simulink model "ROSCO"  (R2022b)
settings: Solver=ode4  StartTime=0.0  StopTime=TMax  FixedStep=simu.dt  RelTol=1e-3  EnableMultiTasking=on
undefined symbols (not defined in the file): DiscIntNeverNeededParam, F, OutList, Parameter, R, rpm2radps, simu, strmatch
libraries: simulink x10
(part 1 of 3)
settings Model: Creator=nabbas  LastModifiedBy=emanu
settings SolverCC: AlgebraicLoopSolver=TrustRegion
settings DataIOCC: SaveTime=off  ReturnWorkspaceOutputs=off  SignalLoggingName=sigsOut
settings OptimizationCC: OptimizeBlockIOStorage=off
settings DebuggingCC: UnconnectedInputMsg=warning  UnconnectedOutputMsg=warning  UnconnectedLineMsg=warning  SFMachineParentedDataDiag=warning  ArithmeticOperatorsInVariantConditions=warning
settings ModelReferenceCC: EnableRefExpFcnMdlSchedulingChecks=on
settings SFSimCC: SimUseLocalCustomCode=off  CustomCodeUndefinedFunction=UseInterfaceOnly
settings RTWCC: RTWUseLocalCustomCode=off  BuildConfiguration=Debug
settings CodeAppCC: ForceParamTrailComments=on  StateflowObjectComments=on  MATLABSourceComments=on

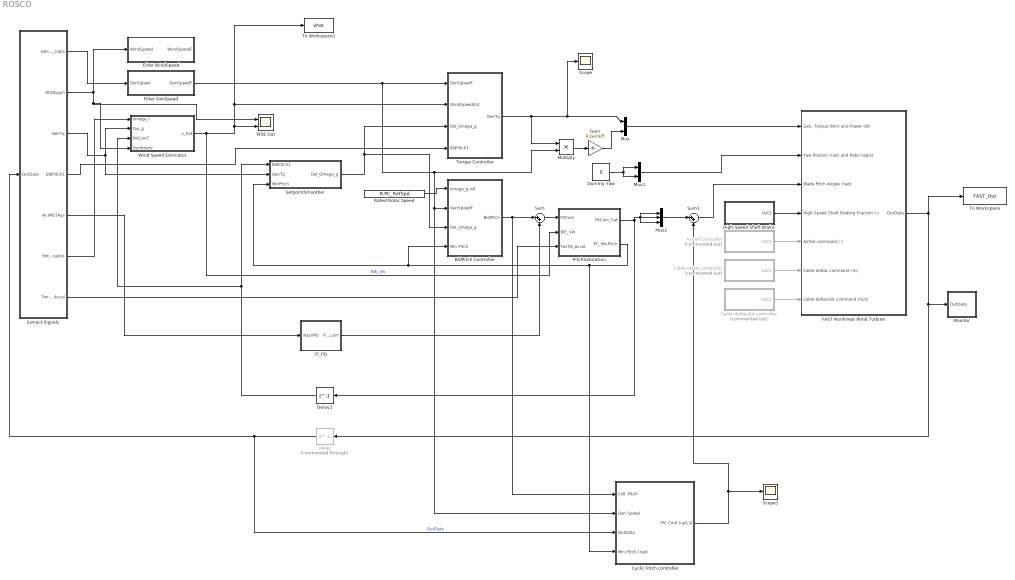
== system ROSCO ==
  AirFoil Controller : Subsystem  Commented=on
  BldPitch Controller : Subsystem
  Cable deltaL controller : Subsystem  Commented=on
  Cable deltaLdot controller : Subsystem  Commented=on
  Cyclic Pitch controller : Subsystem  TreatAsAtomicUnit=on
      settings: MinAlgLoopOccurrences=on
  Delay : Delay  Commented=through  DelayLength=1
  Delay1 : Delay  DelayLength=1
  Dummy Yaw : Constant  Value=0
  Extract Signals : Subsystem  TreatAsAtomicUnit=on
  FAST Nonlinear Wind Turbine : Subsystem  mask(FAST Nonlinear Wind Turbine){}
      mask help: This block contains the FAST S-Function.
      mask init:
      | clear FAST_SFunc
  Filter GenSpeed : Subsystem
  Filter WindSpeed : Subsystem
  Fl_PD : Subsystem
  Gain : Gain  Gain=R.GenEff
  High-Speed Shaft Brake : Subsystem
  Monitor : Subsystem  TreatAsAtomicUnit=on
  Multiply : Product
  Mux : Mux  Inputs=2
  Mux1 : Mux  Inputs=2
  Mux2 : Mux  Inputs=3
  PitchSaturation : Subsystem
  Rated Rotor Speed : Constant  Value=R.PC_RefSpd
  Scope : Scope
  Scope1 : Scope
  SetpointSmoother : Subsystem
  Sum : Sum  Inputs=|++
  Sum1 : Sum  Inputs=|++
  To Workspace : ToWorkspace  VariableName=FAST_Out  SaveFormat=Timeseries  SampleTime=-1
  To Workspace1 : ToWorkspace  VariableName=vhat  SaveFormat=Timeseries  SampleTime=-1
  Torque Controller : Subsystem
  WSE Out : Scope  NumInputPorts=2
  Wind Speed Estimator : Subsystem
  wires:
  FAST Nonlinear Wind Turbine/1(OutData) -> To Workspace/1, Delay/1, Monitor/1(OutData)
  Dummy Yaw/1 -> Mux1/2, Mux1/1
  Mux1/1 -> FAST Nonlinear Wind Turbine/2(Yaw Position (rad) and Rate (rad/s))
  Multiply/1 -> Gain/1
  Extract Signals/1(GenSpeed_rad/s) -> Filter GenSpeed/1(GenSpeed)
  Torque Controller/1(GenTq) -> Scope/1, Mux/1, Multiply/1
  Extract Signals/3(GenTq) -> Wind Speed Estimator/2(tau_g), SetpointSmoother/2(GenTq)
  SetpointSmoother/1(Del_Omega_g) -> BldPitch Controller/3(Del_omega_g), Torque Controller/3(Del_omega_g)
  Rated Rotor Speed/1 -> BldPitch Controller/1(omega_g,ref)
  Gain/1 -> Mux/2
  Extract Signals/2(RtVAvgxh) -> Wind Speed Estimator/4(HorWindV), WSE Out/1, Filter WindSpeed/1(WindSpeed)
  Wind Speed Estimator/1(v_hat) -> PitchSaturation/2(WE_Vw), WSE Out/2, Torque Controller/2(WindSpeedEst), To Workspace1/1  "WE_Vw"
  Delay/1 -> Cyclic Pitch controller/3(OutData), Extract Signals/1(OutData)  "OutData"
  Extract Signals/5(NcIMUTAys) -> Fl_PD/1(NacIMU)
  Fl_PD/1(Fl_Pitcom) -> Sum/2
  Extract Signals/4(BldPitch1) -> Torque Controller/4(BldPitch1)
  Sum/1 -> PitchSaturation/1(PitCom)
  PitchSaturation/1(PitCom_Sat) -> Delay1/1, Mux2/3, Mux2/1, Mux2/2
  PitchSaturation/2(PC_MinPitch) -> Cyclic Pitch controller/4(Min PItch (rad)), BldPitch Controller/4(Min Pitch), SetpointSmoother/3(MinPitch)
  BldPitch Controller/1(BldPitch) -> Cyclic Pitch controller/1(Coll. Pitch), Sum/1
  Extract Signals/6(RotSpeed (rad/s)) -> Wind Speed Estimator/1(omega_r)
  Delay1/1 -> SetpointSmoother/1(BldPitch1), Wind Speed Estimator/3(PitComT)
  Extract Signals/7(TwrFA Accel) -> PitchSaturation/3(TwrFA_Accel)
  Mux/1 -> FAST Nonlinear Wind Turbine/1(Gen. Torque (Nm) and Power (W))
  Filter GenSpeed/1(GenSpeedF) -> Torque Controller/1(GenSpeedF), Multiply/2, BldPitch Controller/2(GenSpeedF), Cyclic Pitch controller/2(Gen Speed)
  Cyclic Pitch controller/1(IPC Cmd (rad,3)) -> Scope1/1, Sum1/2
  Mux2/1 -> Sum1/1
  Sum1/1 -> FAST Nonlinear Wind Turbine/3(Blade Pitch Angles (rad))
  High-Speed Shaft Brake/1(Out1) -> FAST Nonlinear Wind Turbine/4(High-Speed Shaft Braking Fraction (-))
  AirFoil Controller/1(Out1) -> FAST Nonlinear Wind Turbine/5(AirFoil command (-))
  Cable deltaL controller/1(Out1) -> FAST Nonlinear Wind Turbine/6(Cable deltaL command (m))
  Cable deltaLdot controller/1(Out1) -> FAST Nonlinear Wind Turbine/7(Cable deltaLdot command (m/s))

== system ROSCO/AirFoil Controller ==
  Airfoil command : Constant  Value=zeros(1,3)'
  Out1 : Outport
  wires:
  Airfoil command/1 -> Out1/1

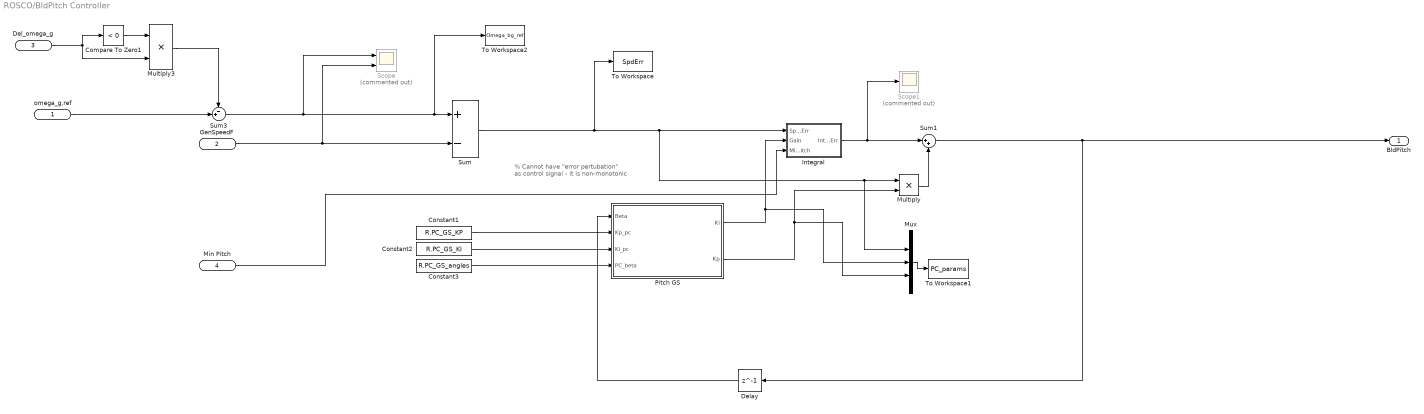
== system ROSCO/BldPitch Controller ==
  note: % Cannot have "error pertubation" as control signal
      | - it is non-monotonic
  omega_g,ref : Inport
  GenSpeedF : Inport  Port=2
  Del_omega_g : Inport  Port=3
  Min Pitch : Inport  Port=4
  Compare To Zero1 : simulink/Logic and Bit Operations/Compare To Zero  relop=<  OutDataTypeStr=boolean
  Constant1 : Constant  Value=R.PC_GS_KP
  Constant2 : Constant  Value=R.PC_GS_KI
  Constant3 : Constant  Value=R.PC_GS_angles
  Delay : Delay  DelayLength=1
  Integral : Subsystem
  Multiply : Product
  Multiply3 : Product
  Mux : Mux  Inputs=5
  Pitch GS : MATLAB Function  TreatAsAtomicUnit=on
  Scope : Scope  Commented=on  NumInputPorts=2
  Scope1 : Scope  Commented=on
  Sum : Sum  Inputs=+-
  Sum1 : Sum  Inputs=|++
  Sum3 : Sum  Inputs=-+|
  To Workspace : ToWorkspace  VariableName=SpdErr  SaveFormat=Timeseries  SampleTime=-1
  To Workspace1 : ToWorkspace  VariableName=PC_params  SaveFormat=Structure  SampleTime=-1
  To Workspace2 : ToWorkspace  VariableName=Omega_bg_ref  SaveFormat=Timeseries  SampleTime=-1
  BldPitch : Outport  VectorParamsAs1DForOutWhenUnconnected=off
  wires:
  Multiply/1 -> Sum1/2
  Integral/1(IntSpdErr) -> Scope1/1, Sum1/1
  Pitch GS/1(Ki) -> Mux/3, Integral/2(Gain)
  Pitch GS/2(Kp) -> Mux/4, Multiply/2
  Mux/1 -> To Workspace1/1
  Sum1/1 -> Delay/1, BldPitch/1
  Sum3/1 -> Scope/1, To Workspace2/1, Sum/1
  GenSpeedF/1 -> Scope/2, Sum/2
  Compare To Zero1/1 -> Multiply3/1
  Del_omega_g/1 -> Compare To Zero1/1, Multiply3/2
  Multiply3/1 -> Sum3/1
  omega_g,ref/1 -> Sum3/2
  Constant1/1 -> Pitch GS/2(Kp_pc)
  Constant2/1 -> Pitch GS/3(Ki_pc)
  Constant3/1 -> Pitch GS/4(PC_beta)
  Delay/1 -> Pitch GS/1(Beta)
  Min Pitch/1 -> Integral/3(Min Pitch)
  Sum/1 -> To Workspace/1, Mux/2, Multiply/1, Integral/1(SpeedErr)

== system ROSCO/Cable deltaL controller ==
  Cable deltaL command : Constant  Value=zeros(1,20)'
  Out1 : Outport
  wires:
  Cable deltaL command/1 -> Out1/1

== system ROSCO/Cable deltaLdot controller ==
  Cable deltaLdot command : Constant  Value=zeros(1,20)'
  Out1 : Outport
  wires:
  Cable deltaLdot command/1 -> Out1/1

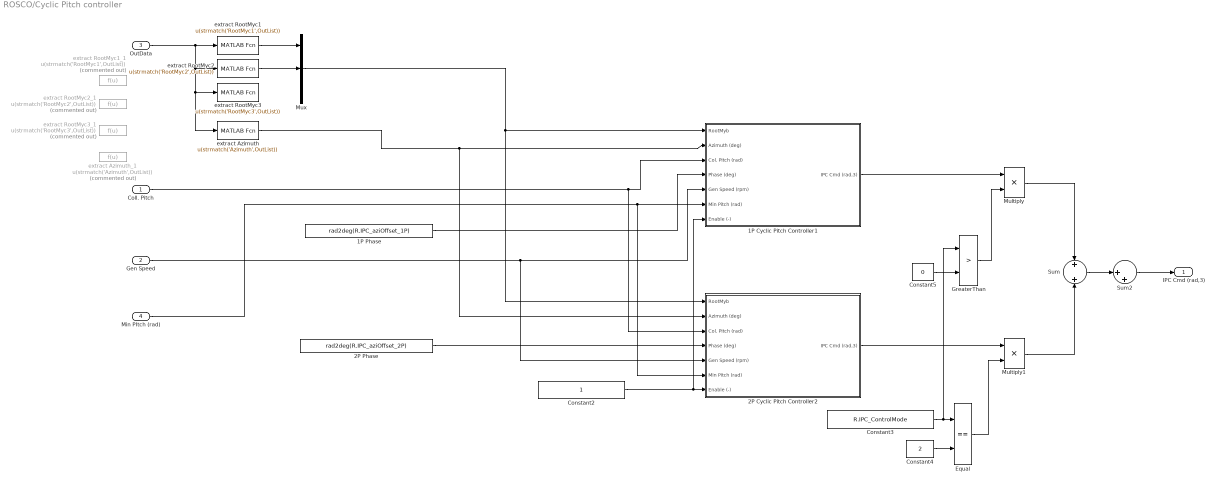
== system ROSCO/Cyclic Pitch controller ==
  Coll. Pitch : Inport
  Gen Speed : Inport  Port=2
  OutData : Inport  Port=3
  Min PItch (rad) : Inport  Port=4
  1P Cyclic Pitch Controller1 : Subsystem
  1P Phase : Constant  Value=rad2deg(R.IPC_aziOffset_1P)
  2P Cyclic Pitch Controller2 : Subsystem
  2P Phase : Constant  Value=rad2deg(R.IPC_aziOffset_2P)
  Constant2 : Constant
  Constant3 : Constant  Value=R.IPC_ControlMode
  Constant4 : Constant  Value=2
  Constant5 : Constant  Value=0
  Equal : RelationalOperator  Operator===  OutDataTypeStr=boolean  RndMeth=Simplest  InputSameDT=off
  GreaterThan : RelationalOperator  Operator=>  OutDataTypeStr=boolean  RndMeth=Simplest  InputSameDT=off
  Multiply : Product
  Multiply1 : Product
  Mux : Mux  Inputs=3
  Sum : Sum  Inputs=+|+
  Sum2 : Sum  Inputs=|++
  extract Azimuth : MATLABFcn  MATLABFcn=u(strmatch('Azimuth',OutList))
  extract Azimuth_1 : Fcn  Commented=on  Expr=u(strmatch('Azimuth',OutList))
  extract RootMyc1 : MATLABFcn  MATLABFcn=u(strmatch('RootMyc1',OutList))
  extract RootMyc1_1 : Fcn  Commented=on  Expr=u(strmatch('RootMyc1',OutList))
  extract RootMyc2 : MATLABFcn  MATLABFcn=u(strmatch('RootMyc2',OutList))
  extract RootMyc2_1 : Fcn  Commented=on  Expr=u(strmatch('RootMyc2',OutList))
  extract RootMyc3 : MATLABFcn  MATLABFcn=u(strmatch('RootMyc3',OutList))
  extract RootMyc3_1 : Fcn  Commented=on  Expr=u(strmatch('RootMyc3',OutList))
  IPC Cmd (rad,3) : Outport  VectorParamsAs1DForOutWhenUnconnected=off
  wires:
  1P Phase/1 -> 1P Cyclic Pitch Controller1/4(Phase (deg))
  Coll. Pitch/1 -> 2P Cyclic Pitch Controller2/3(Col. Pitch (rad)), 1P Cyclic Pitch Controller1/3(Col. Pitch (rad))
  Gen Speed/1 -> 2P Cyclic Pitch Controller2/5(Gen Speed (rpm)), 1P Cyclic Pitch Controller1/5(Gen Speed (rpm))
  1P Cyclic Pitch Controller1/1(IPC Cmd (rad,3)) -> Multiply/1
  extract RootMyc1/1 -> Mux/1
  extract RootMyc2/1 -> Mux/2
  ? -> Mux/3
  Mux/1 -> 1P Cyclic Pitch Controller1/1(RootMyb), 2P Cyclic Pitch Controller2/1(RootMyb)
  extract Azimuth/1 -> 2P Cyclic Pitch Controller2/2(Azimuth (deg)), 1P Cyclic Pitch Controller1/2(Azimuth (deg))
  Min PItch (rad)/1 -> 2P Cyclic Pitch Controller2/6(Min Pitch (rad)), 1P Cyclic Pitch Controller1/6(Min Pitch (rad))
  2P Phase/1 -> 2P Cyclic Pitch Controller2/4(Phase (deg))
  2P Cyclic Pitch Controller2/1(IPC Cmd (rad,3)) -> Multiply1/1
  Multiply1/1 -> Sum/2
  Multiply/1 -> Sum/1
  OutData/1 -> extract RootMyc1/1, extract RootMyc2/1, extract RootMyc3/1, extract Azimuth/1
  Sum/1 -> Sum2/1
  Sum2/1 -> IPC Cmd (rad,3)/1
  Constant2/1 -> 1P Cyclic Pitch Controller1/7(Enable (-)), 2P Cyclic Pitch Controller2/7(Enable (-))
  Constant4/1 -> Equal/2
  Equal/1 -> Multiply1/2
  Constant3/1 -> GreaterThan/1, Equal/1
  Constant5/1 -> GreaterThan/2
  GreaterThan/1 -> Multiply/2

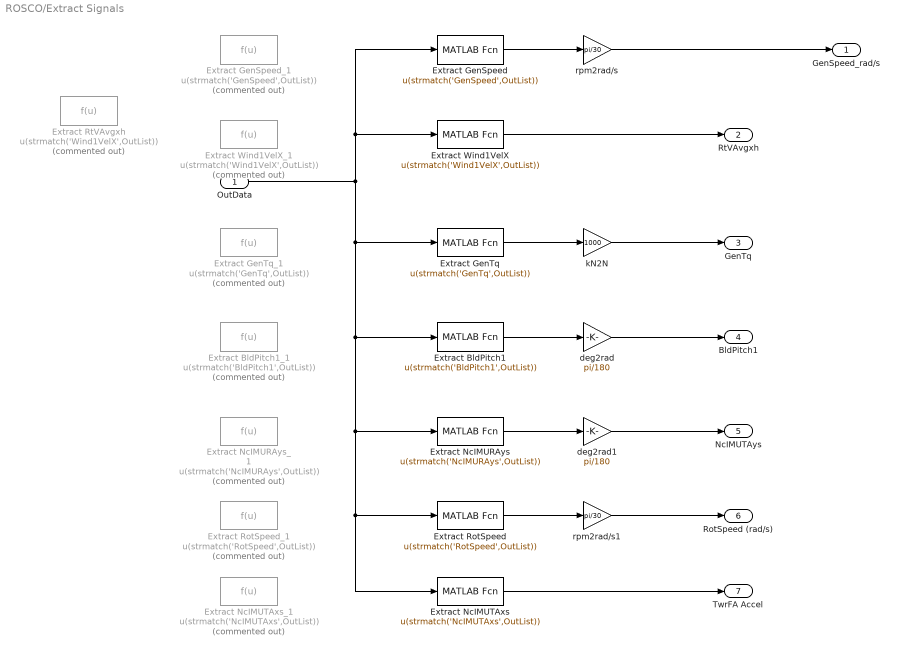
== system ROSCO/Extract Signals ==
  OutData : Inport
  Extract BldPitch1 : MATLABFcn  MATLABFcn=u(strmatch('BldPitch1',OutList))
  Extract BldPitch1_1 : Fcn  Commented=on  Expr=u(strmatch('BldPitch1',OutList))
  Extract GenSpeed : MATLABFcn  MATLABFcn=u(strmatch('GenSpeed',OutList))
  Extract GenSpeed_1 : Fcn  Commented=on  Expr=u(strmatch('GenSpeed',OutList))
  Extract GenTq : MATLABFcn  MATLABFcn=u(strmatch('GenTq',OutList))
  Extract GenTq_1 : Fcn  Commented=on  Expr=u(strmatch('GenTq',OutList))
  Extract NcIMURAys : MATLABFcn  MATLABFcn=u(strmatch('NcIMURAys',OutList))
  Extract NcIMURAys_1 : Fcn  Commented=on  Expr=u(strmatch('NcIMURAys',OutList))
  Extract NcIMUTAxs : MATLABFcn  MATLABFcn=u(strmatch('NcIMUTAxs',OutList))
  Extract NcIMUTAxs_1 : Fcn  Commented=on  Expr=u(strmatch('NcIMUTAxs',OutList))
  Extract RotSpeed : MATLABFcn  MATLABFcn=u(strmatch('RotSpeed',OutList))
  Extract RotSpeed_1 : Fcn  Commented=on  Expr=u(strmatch('RotSpeed',OutList))
  Extract RtVAvgxh : Fcn  Commented=on  Expr=u(strmatch('Wind1VelX',OutList))
  Extract Wind1VelX : MATLABFcn  MATLABFcn=u(strmatch('Wind1VelX',OutList))
  Extract Wind1VelX_1 : Fcn  Commented=on  Expr=u(strmatch('Wind1VelX',OutList))
  deg2rad : Gain  Gain=pi/180
  deg2rad1 : Gain  Gain=pi/180
  kN2N : Gain  Gain=1000
  rpm2rad/s : Gain  Gain=pi/30
  rpm2rad/s1 : Gain  Gain=pi/30
  GenSpeed_rad/s : Outport  VectorParamsAs1DForOutWhenUnconnected=off
  RtVAvgxh : Outport  Port=2  VectorParamsAs1DForOutWhenUnconnected=off
  GenTq : Outport  Port=3  VectorParamsAs1DForOutWhenUnconnected=off
  BldPitch1 : Outport  Port=4  VectorParamsAs1DForOutWhenUnconnected=off
  NcIMUTAys : Outport  Port=5  VectorParamsAs1DForOutWhenUnconnected=off
  RotSpeed (rad/s) : Outport  Port=6  VectorParamsAs1DForOutWhenUnconnected=off
  TwrFA Accel : Outport  Port=7  VectorParamsAs1DForOutWhenUnconnected=off
  wires:
  OutData/1 -> Extract GenSpeed/1, Extract Wind1VelX/1, Extract GenTq/1, Extract BldPitch1/1, Extract NcIMURAys/1, Extract NcIMUTAxs/1, Extract RotSpeed/1
  Extract Wind1VelX/1 -> RtVAvgxh/1
  Extract GenSpeed/1 -> rpm2rad/s/1
  Extract BldPitch1/1 -> deg2rad/1
  deg2rad/1 -> BldPitch1/1
  Extract GenTq/1 -> kN2N/1
  kN2N/1 -> GenTq/1
  Extract NcIMURAys/1 -> deg2rad1/1
  deg2rad1/1 -> NcIMUTAys/1
  Extract RotSpeed/1 -> rpm2rad/s1/1
  rpm2rad/s1/1 -> RotSpeed (rad/s)/1
  Extract NcIMUTAxs/1 -> TwrFA Accel/1
  rpm2rad/s/1 -> GenSpeed_rad/s/1

== system ROSCO/FAST Nonlinear Wind Turbine ==
  note: 43
  Gen. Torque (Nm) and Power (W) : Inport
  Yaw Position (rad) and Rate (rad/s) : Inport  Port=2
  Blade Pitch Angles (rad) : Inport  Port=3
  High-Speed Shaft Braking Fraction (-) : Inport  Port=4
  AirFoil command (-) : Inport  Port=5
  Cable deltaL command (m) : Inport  Port=6
  Cable deltaLdot command (m/s) : Inport  Port=7
  Mux1 : Mux
  S-Function : S-Function  FunctionName=FAST_SFunc  Parameters=FAST_InputFileName, TMax, 0  SFunctionDeploymentMode=off  EnableBusSupport=off
  Signal Specification1 : SignalSpecification  OutDataTypeStr=double  Dimensions=2
  Signal Specification2 : SignalSpecification  OutDataTypeStr=double  Dimensions=2
  OutData : Outport
  wires:
  Gen. Torque (Nm) and Power (W)/1 -> Signal Specification1/1
  S-Function/1 -> OutData/1
  Mux1/1 -> S-Function/1
  Blade Pitch Angles (rad)/1 -> Mux1/3
  Yaw Position (rad) and Rate (rad/s)/1 -> Signal Specification2/1
  Signal Specification1/1 -> Mux1/1
  Signal Specification2/1 -> Mux1/2
  High-Speed Shaft Braking Fraction (-)/1 -> Mux1/4

== system ROSCO/Filter GenSpeed ==
  GenSpeed : Inport
  Discrete Filter : DiscreteFilter  Numerator=F.HSS.b  Denominator=F.HSS.a  InitialStates=R.VS_RefSpd/(sum(F.HSS.a(2:end))+1)
  Scope : Scope  NumInputPorts=2
  To Workspace2 : ToWorkspace  VariableName=Om_f  SaveFormat=Timeseries  SampleTime=-1
  GenSpeedF : Outport  VectorParamsAs1DForOutWhenUnconnected=off
  wires:
  Discrete Filter/1 -> Scope/2, To Workspace2/1, GenSpeedF/1
  GenSpeed/1 -> Scope/1, Discrete Filter/1

== system ROSCO/Filter WindSpeed ==
  WindSpeed : Inport
  Discrete Filter : DiscreteFilter  Numerator=F.Wind.b  Denominator=F.Wind.a  InitialStates=10
  To Workspace2 : ToWorkspace  VariableName=WindSpeedF  SaveFormat=Timeseries  SampleTime=-1
  WindSpeedF : Outport  VectorParamsAs1DForOutWhenUnconnected=off
  wires:
  Discrete Filter/1 -> WindSpeedF/1, To Workspace2/1
  WindSpeed/1 -> Discrete Filter/1

== system ROSCO/Fl_PD ==
  NacIMU : Inport
  Constant : Constant
  Enable : Gain  Gain=R.Fl_Mode
  Fl_HPF : DiscreteFilter  Numerator=F.F_Fl_HPF.b  Denominator=F.F_Fl_HPF.b
  Fl_LPF : DiscreteFilter  Numerator=F.F_Fl.b  Denominator=F.F_Fl.a
  Gain1 : Gain  Gain=-R.Fl_Kp
  Integral : Subsystem
  Scope : Scope
  Fl_Pitcom : Outport
  wires:
  Constant/1 -> Integral/2(Gain)
  NacIMU/1 -> Fl_LPF/1  "FA_AccR"
  Integral/1(Int x) -> Gain1/1
  Fl_HPF/1 -> Integral/1(x)  "FA_AccF"
  Gain1/1 -> Enable/1  "Fl_Pitcom"
  Enable/1 -> Scope/1, Fl_Pitcom/1  "Fl_Pitcom"
  Fl_LPF/1 -> Fl_HPF/1  "FA_AccF"

== system ROSCO/High-Speed Shaft Brake ==
  High-Speed Shaft Braking Fraction : Constant  Value=0
  Out1 : Outport
  wires:
  High-Speed Shaft Braking Fraction/1 -> Out1/1

== system ROSCO/Monitor ==
  OutData : Inport
  Extract BldPitch1 : Fcn  Expr=u(strmatch('BldPitch1',OutList))
  Extract GenTq : Fcn  Expr=u(strmatch('GenTq',OutList))
  Extract RotSpeed : Fcn  Expr=u(strmatch('RotSpeed',OutList))
  Scope : Scope  NumInputPorts=3
  wires:
  Extract BldPitch1/1 -> Scope/3
  OutData/1 -> Extract RotSpeed/1, Extract BldPitch1/1, Extract GenTq/1
  Extract RotSpeed/1 -> Scope/1
  Extract GenTq/1 -> Scope/2

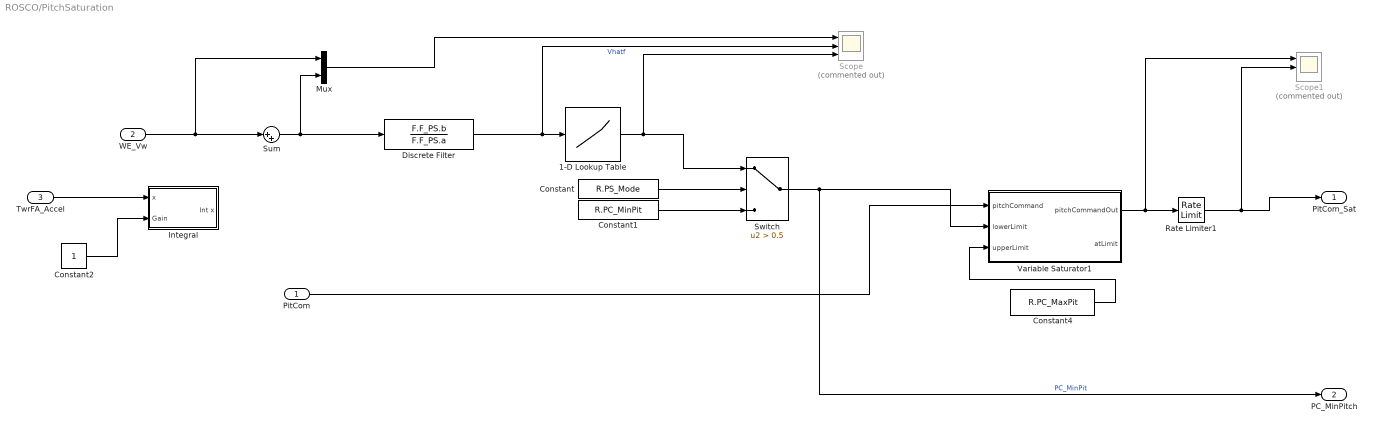
== system ROSCO/PitchSaturation ==
  PitCom : Inport
  WE_Vw : Inport  Port=2
  TwrFA_Accel : Inport  Port=3
  1-D Lookup Table : Lookup_n-D  NumberOfTableDimensions=1  BreakpointsForDimension1=R.PS_WindSpeeds  Table=R.PS_BldPitchMin  InternalRulePriority=Speed  RndMeth=Simplest
  Constant : Constant  Value=R.PS_Mode
  Constant1 : Constant  Value=R.PC_MinPit
  Constant2 : Constant
  Constant4 : Constant  Value=R.PC_MaxPit
  Discrete Filter : DiscreteFilter  Numerator=F.F_PS.b  Denominator=F.F_PS.a  InitialStates=R.WE_v0/(sum(F.F_PS.a(2:end))+1)
  Integral : Subsystem
  Mux : Mux  Inputs=2
  Rate Limiter1 : RateLimiter  RisingSlewLimit=R.PC_MaxRat  FallingSlewLimit=-R.PC_MaxRat  SampleTimeMode=inherited
  Scope : Scope  Commented=on  NumInputPorts=3
  Scope1 : Scope  Commented=on  NumInputPorts=3
  Sum : Sum  Inputs=|++
  Switch : Switch  Criteria=u2 > Threshold  Threshold=0.5  SaturateOnIntegerOverflow=off  InputSameDT=off
  Variable Saturator1 : MATLAB Function  TreatAsAtomicUnit=on
  PitCom_Sat : Outport
  PC_MinPitch : Outport  Port=2
  wires:
  1-D Lookup Table/1 -> Scope/3, Switch/1
  Constant/1 -> Switch/2
  Discrete Filter/1 -> Scope/2, 1-D Lookup Table/1  "Vhatf"
  Constant1/1 -> Switch/3
  Switch/1 -> PC_MinPitch/1, Variable Saturator1/2(lowerLimit)  "PC_MinPit"
  Constant4/1 -> Variable Saturator1/3(upperLimit)
  Variable Saturator1/1(pitchCommandOut) -> Scope1/1, Rate Limiter1/1
  Rate Limiter1/1 -> Scope1/2, PitCom_Sat/1
  PitCom/1 -> Variable Saturator1/1(pitchCommand)
  TwrFA_Accel/1 -> Integral/1(x)
  Constant2/1 -> Integral/2(Gain)
  WE_Vw/1 -> Mux/1, Sum/1
  Sum/1 -> Mux/2, Discrete Filter/1
  Mux/1 -> Scope/1

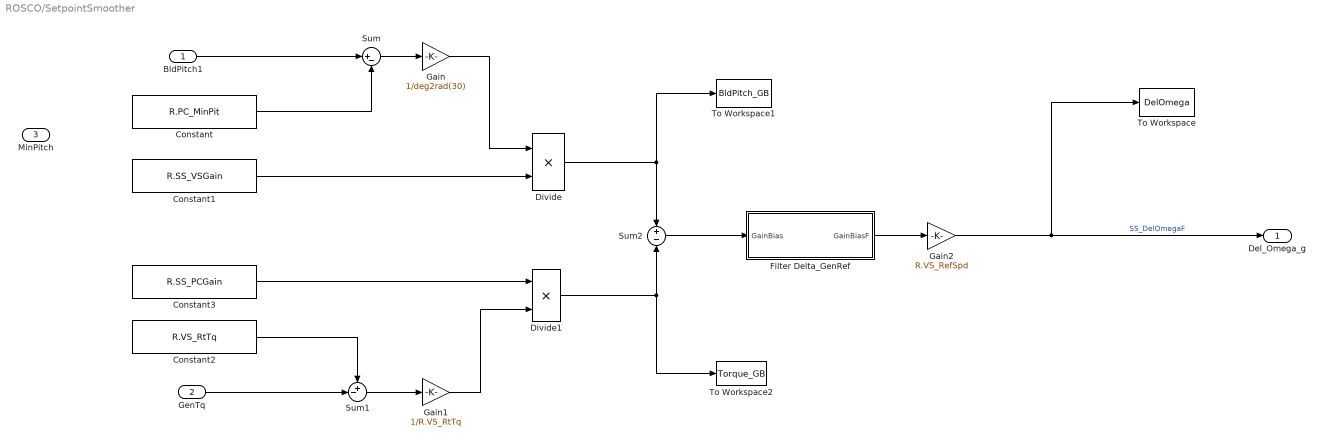
== system ROSCO/SetpointSmoother ==
  BldPitch1 : Inport
  GenTq : Inport  Port=2
  MinPitch : Inport  Port=3
  Constant : Constant  Value=R.PC_MinPit
  Constant1 : Constant  Value=R.SS_VSGain
  Constant2 : Constant  Value=R.VS_RtTq
  Constant3 : Constant  Value=R.SS_PCGain
  Divide : Product  Inputs=**
  Divide1 : Product  Inputs=**
  Filter Delta_GenRef : Subsystem
  Gain : Gain  Gain=1/deg2rad(30)
  Gain1 : Gain  Gain=1/R.VS_RtTq
  Gain2 : Gain  Gain=R.VS_RefSpd
  Sum : Sum  Inputs=|+-
  Sum1 : Sum  Inputs=+-|
  Sum2 : Sum  Inputs=+|-
  To Workspace : ToWorkspace  VariableName=DelOmega  SaveFormat=Timeseries  SampleTime=-1
  To Workspace1 : ToWorkspace  VariableName=BldPitch_GB  SaveFormat=Timeseries  SampleTime=-1
  To Workspace2 : ToWorkspace  VariableName=Torque_GB  SaveFormat=Timeseries  SampleTime=-1
  Del_Omega_g : Outport  VectorParamsAs1DForOutWhenUnconnected=off
  wires:
  Divide1/1 -> Sum2/2, To Workspace2/1
  Divide/1 -> Sum2/1, To Workspace1/1
  Filter Delta_GenRef/1(GainBiasF) -> Gain2/1
  Constant3/1 -> Divide1/1
  Constant1/1 -> Divide/2
  Sum/1 -> Gain/1
  BldPitch1/1 -> Sum/1
  Sum2/1 -> Filter Delta_GenRef/1(GainBias)
  Constant2/1 -> Sum1/1
  Sum1/1 -> Gain1/1
  GenTq/1 -> Sum1/2
  Gain/1 -> Divide/1
  Gain1/1 -> Divide1/2
  Gain2/1 -> To Workspace/1, Del_Omega_g/1  "SS_DelOmegaF"
  Constant/1 -> Sum/2

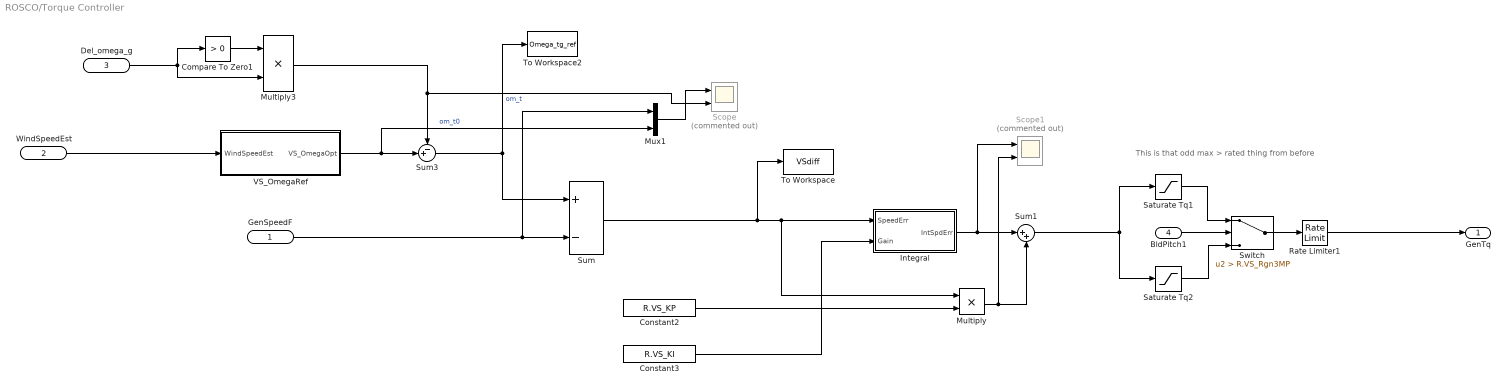
== system ROSCO/Torque Controller ==
  note: This is that odd max > rated thing from before
  GenSpeedF : Inport
  WindSpeedEst : Inport  Port=2
  Del_omega_g : Inport  Port=3
  BldPitch1 : Inport  Port=4
  Compare To Zero1 : simulink/Logic and Bit Operations/Compare To Zero  relop=>  OutDataTypeStr=boolean
  Constant2 : Constant  Value=R.VS_KP
  Constant3 : Constant  Value=R.VS_KI
  Integral : Subsystem
  Multiply : Product
  Multiply3 : Product
  Mux1 : Mux  Inputs=2
  Rate Limiter1 : RateLimiter  RisingSlewLimit=R.VS_MaxRat  FallingSlewLimit=-R.VS_MaxRat  SampleTimeMode=inherited  InitialCondition=R.VS_RtTq
  Saturate Tq1 : Saturate  UpperLimit=R.VS_RtTq  LowerLimit=0
  Saturate Tq2 : Saturate  UpperLimit=R.VS_RtTq  LowerLimit=0
  Scope : Scope  Commented=on  NumInputPorts=2
  Scope1 : Scope  Commented=on  NumInputPorts=2
  Sum : Sum  Inputs=+-
  Sum1 : Sum  Inputs=|++
  Sum3 : Sum  Inputs=-+|
  Switch : Switch  Criteria=u2 > Threshold  Threshold=R.VS_Rgn3MP  SaturateOnIntegerOverflow=off  InputSameDT=off
  To Workspace : ToWorkspace  VariableName=VSdiff  SaveFormat=Timeseries  SampleTime=-1
  To Workspace2 : ToWorkspace  VariableName=Omega_tg_ref  SaveFormat=Timeseries  SampleTime=-1
  VS_OmegaRef : Subsystem
  GenTq : Outport  VectorParamsAs1DForOutWhenUnconnected=off
  wires:
  Multiply/1 -> Scope1/2, Sum1/2
  Integral/1(IntSpdErr) -> Scope1/1, Sum1/1
  Constant2/1 -> Multiply/2
  Constant3/1 -> Integral/2(Gain)
  VS_OmegaRef/1(VS_OmegaOpt) -> Mux1/2, Sum3/2  "om_t0"
  GenSpeedF/1 -> Mux1/1, Sum/2
  Sum3/1 -> To Workspace2/1, Sum/1  "om_t"
  Saturate Tq2/1 -> Switch/3
  Switch/1 -> Rate Limiter1/1
  Saturate Tq1/1 -> Switch/1
  BldPitch1/1 -> Switch/2
  Compare To Zero1/1 -> Multiply3/1
  Del_omega_g/1 -> Compare To Zero1/1, Multiply3/2
  Multiply3/1 -> Scope/2, Sum3/1
  Mux1/1 -> Scope/1
  Sum1/1 -> Saturate Tq2/1, Saturate Tq1/1
  Rate Limiter1/1 -> GenTq/1
  Sum/1 -> To Workspace/1, Integral/1(SpeedErr), Multiply/1
  WindSpeedEst/1 -> VS_OmegaRef/1(WindSpeedEst)

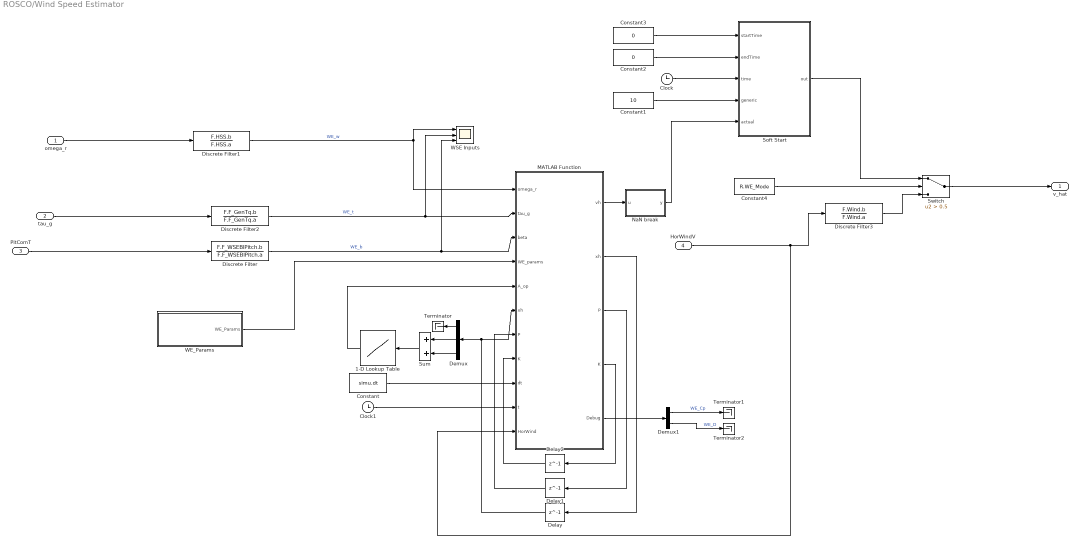
== system ROSCO/Wind Speed Estimator ==
  omega_r : Inport
  tau_g : Inport  Port=2
  PitComT : Inport  Port=3
  HorWindV : Inport  Port=4
  1-D Lookup Table : Lookup_n-D  NumberOfTableDimensions=1  BreakpointsForDimension1=[-5:5]  Table=tanh([-5:5])  InternalRulePriority=Speed  RndMeth=Simplest
  Clock : Clock
  Clock1 : Clock
  Constant : Constant  Value=simu.dt
  Constant1 : Constant  Value=10
  Constant2 : Constant  Value=0
  Constant3 : Constant  Value=0
  Constant4 : Constant  Value=R.WE_Mode
  Delay : Delay  DelayLength=1  InitialCondition=[R.WE_GearboxRatio, 0, R.WE_v0]'
  Delay1 : Delay  DelayLength=1  InitialCondition=diag([0.1, 0.1, 1])^2
  Delay2 : Delay  DelayLength=1  InitialCondition=zeros(3,1)
  Demux : Demux  Outputs=3
  Demux1 : Demux  Outputs=2
  Discrete Filter : DiscreteFilter  Numerator=F.F_WSEBlPitch.b  Denominator=F.F_WSEBlPitch.a
  Discrete Filter1 : DiscreteFilter  Numerator=F.HSS.b  Denominator=F.HSS.a  InitialStates=R.VS_RefSpd/(sum(F.HSS.a(2:end))+1)/R.GBRatio
  Discrete Filter2 : DiscreteFilter  Numerator=F.F_GenTq.b  Denominator=F.F_GenTq.a  InitialStates=R.VS_RtTq/(sum(F.F_GenTq.a(2:end))+1)
  Discrete Filter3 : DiscreteFilter  Numerator=F.Wind.b  Denominator=F.Wind.a  InitialStates=10
  MATLAB Function : MATLAB Function  TreatAsAtomicUnit=on
  NaN break : MATLAB Function  TreatAsAtomicUnit=on
  Soft Start : MATLAB Function  TreatAsAtomicUnit=on
  Sum : Sum
  Switch : Switch  Criteria=u2 > Threshold  Threshold=0.5  SaturateOnIntegerOverflow=off  InputSameDT=off
  Terminator : Terminator
  Terminator1 : Terminator
  Terminator2 : Terminator
  WE_Params : Subsystem
  WSE Inputs : Scope  NumInputPorts=3
  v_hat : Outport  VectorParamsAs1DForOutWhenUnconnected=off
  wires:
  MATLAB Function/2(xh) -> Delay/1
  Delay/1 -> Demux/1, MATLAB Function/6("xh ")
  MATLAB Function/3(P) -> Delay1/1
  Delay1/1 -> MATLAB Function/7("P ")
  omega_r/1 -> Discrete Filter1/1
  tau_g/1 -> Discrete Filter2/1
  MATLAB Function/4(K) -> Delay2/1
  Delay2/1 -> MATLAB Function/8("K ")
  Constant/1 -> MATLAB Function/9(dt)
  Demux/2 -> Sum/1
  Demux/3 -> Sum/2
  Demux/1 -> Terminator/1
  Sum/1 -> 1-D Lookup Table/1
  1-D Lookup Table/1 -> MATLAB Function/5(A_op)
  WE_Params/1(WE_Params) -> MATLAB Function/4(WE_params)
  Clock/1 -> Soft Start/3(time)
  Constant1/1 -> Soft Start/4(generic)
  Constant2/1 -> Soft Start/2(endTime)
  Constant3/1 -> Soft Start/1(startTime)
  MATLAB Function/1(vh) -> NaN break/1(u)
  Discrete Filter/1 -> WSE Inputs/3, MATLAB Function/3(beta)  "WE_b"
  Discrete Filter1/1 -> MATLAB Function/1(omega_r), WSE Inputs/1  "WE_w"
  Discrete Filter2/1 -> MATLAB Function/2(tau_g), WSE Inputs/2  "WE_t"
  PitComT/1 -> Discrete Filter/1
  Soft Start/1(out) -> Switch/1
  Switch/1 -> v_hat/1
  HorWindV/1 -> MATLAB Function/11(HorWind), Discrete Filter3/1
  Constant4/1 -> Switch/2
  MATLAB Function/5(Debug) -> Demux1/1
  Demux1/1 -> Terminator1/1  "WE_Cp"
  Demux1/2 -> Terminator2/1  "WE_D"
  Clock1/1 -> MATLAB Function/10(t)
  Discrete Filter3/1 -> Switch/3
  NaN break/1(y) -> Soft Start/5(actual)

== system ROSCO/BldPitch Controller/Integral ==
  SpeedErr : Inport
  Gain : Inport  Port=2
  Min Pitch : Inport  Port=3
  Gain1 : Gain  Gain=simu.dt
  Maximum Pitch : Constant  Value=R.PC_MaxPit
  Minimum Pitch : Constant  Value=R.PC_MinPit
  Multiply : Product
  Saturate Integral Term : simulink/Discontinuities/Saturation Dynamic  OutMin=[]  OutMax=[]  OutDataTypeStr=Inherit: Same as second input  OutDataType=fixdt(1, 16)  OutScaling=2^-10  RndMeth=Nearest  DoSatur=off
  Sum : Sum  Inputs=|++
  Unit Delay : UnitDelay  SampleTime=-1  HasFrameUpgradeWarning=on
  IntSpdErr : Outport  VectorParamsAs1DForOutWhenUnconnected=off
  wires:
  Maximum Pitch/1 -> Saturate Integral Term/1
  Unit Delay/1 -> Sum/2
  Sum/1 -> Saturate Integral Term/2
  SpeedErr/1 -> Gain1/1
  Gain/1 -> Multiply/2
  Saturate Integral Term/1 -> IntSpdErr/1, Unit Delay/1
  Gain1/1 -> Multiply/1
  Multiply/1 -> Sum/1
  Min Pitch/1 -> Saturate Integral Term/3

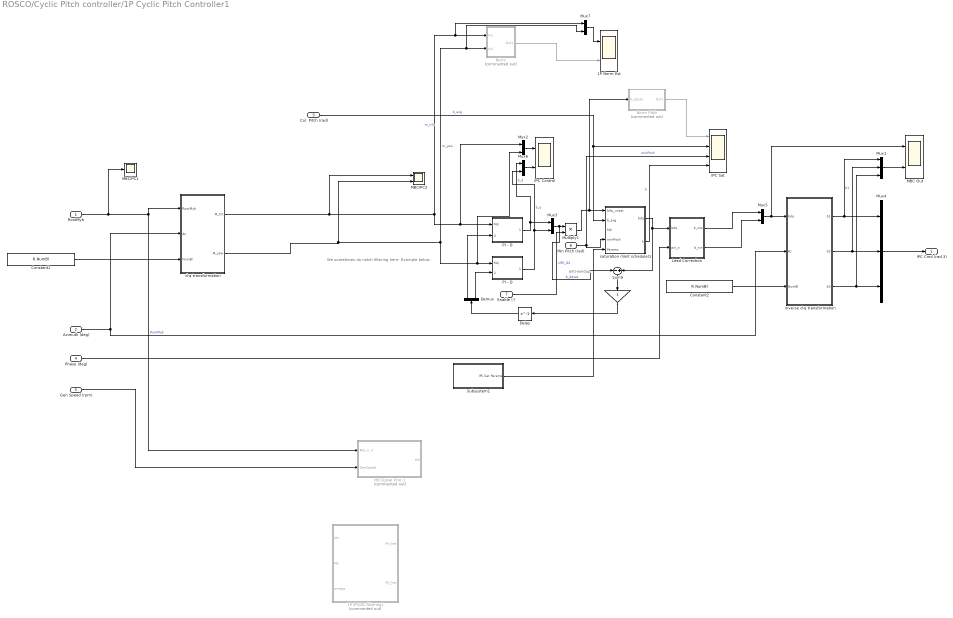
== system ROSCO/Cyclic Pitch controller/1P Cyclic Pitch Controller1 ==
  note: We sometimes do notch filtering here. Example below.
  note: k
  note: anti-windup
  RootMyb : Inport
  Azimuth (deg) : Inport  Port=2
  Col. Pitch (rad) : Inport  Port=3
  Phase (deg) : Inport  Port=4
  Gen Speed (rpm) : Inport  Port=5
  Min Pitch (rad) : Inport  Port=6
  Enable (-) : Inport  Port=7
  " " : Gain
  1P IPCDQ Filtering1 : Subsystem  Commented=on
  1P Norm Est : Scope  NumInputPorts=2
  Constant1 : Constant  Value=R.NumBl
  Constant2 : Constant  Value=R.NumBl
  Delay : Delay  DelayLength=1
  Demux : Demux  Outputs=2
  IPC Control : Scope  NumInputPorts=2
  IPC Sat : Scope  NumInputPorts=4
  Lead Correction : MATLAB Function  TreatAsAtomicUnit=on
  M0 Signal Proc.1 : Subsystem  Commented=on
  MBC Out : Scope  NumInputPorts=2
  MBCIPC1 : Scope
  MBCIPC2 : Scope  NumInputPorts=2
  Multiply1 : Product
  Mux1 : Mux  Inputs=3
  Mux{2..3,5..7} (5 alike) : Mux  Inputs=2
  Mux4 : Mux  Inputs=3
  Norm : Subsystem  Commented=on
  Norm Pitch : Subsystem  Commented=on
  PI - D : Subsystem  TreatAsAtomicUnit=on  SystemSampleTime=simu.dt
      settings: MinAlgLoopOccurrences=on
  PI - Q : Subsystem  TreatAsAtomicUnit=on  SystemSampleTime=simu.dt
      settings: MinAlgLoopOccurrences=on
  Subsystem1 : Subsystem
  Sum9 : Sum  Inputs=-|+
  d-q transformation : MATLAB Function  TreatAsAtomicUnit=on
  inverse d-q transformation : MATLAB Function  TreatAsAtomicUnit=on
  saturation (limit schedule)1 : MATLAB Function  TreatAsAtomicUnit=on
  IPC Cmd (rad,3) : Outport  VectorParamsAs1DForOutWhenUnconnected=off
  wires:
  Col. Pitch (rad)/1 -> saturation (limit schedule)1/2(b_avg), IPC Sat/2  "b_avg"
  saturation (limit schedule)1/1(bdq) -> Sum9/2, Lead Correction/1(bdq)
  Gen Speed (rpm)/1 -> M0 Signal Proc.1/2(GenSpeed)
  d-q transformation/1(M_tilt) -> Mux2/1, PI - D/1(Md), Mux7/1, Norm/1(In1), MBCIPC2/1  "m_tilt"
  Mux5/1 -> MBC Out/1, inverse d-q transformation/1(bdq)
  inverse d-q transformation/3(b3) -> Mux1/3, Mux4/3
  Phase (deg)/1 -> Lead Correction/2(psi_o)
  PI - Q/1(Theta_yaw) -> Mux6/2, Mux3/2  "b_q"
  PI - D/1(Theta_tilt) -> Mux3/1, Mux6/1  "b_d"
  Demux/1 -> PI - D/2(Anti-windup)
  inverse d-q transformation/1(b1) -> Mux1/1, Mux4/1  "b1"
  Demux/2 -> PI - Q/2(Anti-windup)
  inverse d-q transformation/2(b2) -> Mux1/2, Mux4/2
  Mux4/1 -> IPC Cmd (rad,3)/1
  Delay/1 -> Demux/1
  " "/1 -> Delay/1
  RootMyb/1 -> M0 Signal Proc.1/1("My1,2, 3"), d-q transformation/1(RootMyb), MBCIPC1/1  "RootMyb"
  Sum9/1 -> " "/1
  Azimuth (deg)/1 -> d-q transformation/2(Az), inverse d-q transformation/2(Az)
  Lead Correction/1(b_cos) -> Mux5/1
  Lead Correction/2(b_sin) -> Mux5/2
  saturation (limit schedule)1/2(k) -> IPC Sat/4
  Constant1/1 -> d-q transformation/3(NumBl)
  Constant2/1 -> inverse d-q transformation/3(NumBl)
  d-q transformation/2(M_yaw) -> Mux2/2, PI - Q/1(Mq), Mux7/2, Norm/2(In2), MBCIPC2/2  "m_yaw"
  Mux1/1 -> MBC Out/2
  Mux6/1 -> IPC Control/2
  Mux2/1 -> IPC Control/1
  Mux7/1 -> 1P Norm Est/1
  Norm/1(Out1) -> 1P Norm Est/2
  Min Pitch (rad)/1 -> IPC Sat/3, saturation (limit schedule)1/4(minPitch)  "minPitch"
  Norm Pitch/1(Out1) -> IPC Sat/1
  Enable (-)/1 -> Multiply1/2  "cIPC_GS"
  Subsystem1/1(IPC Sat Params) -> saturation (limit schedule)1/5(Params)
  Mux3/1 -> Sum9/1, Multiply1/1  "b_dqsat"
  Multiply1/1 -> Norm Pitch/1(b_dqsat), saturation (limit schedule)1/1(bdq_unsat)
  ? -> 1P IPCDQ Filtering1/2(My)  "m_yaw"

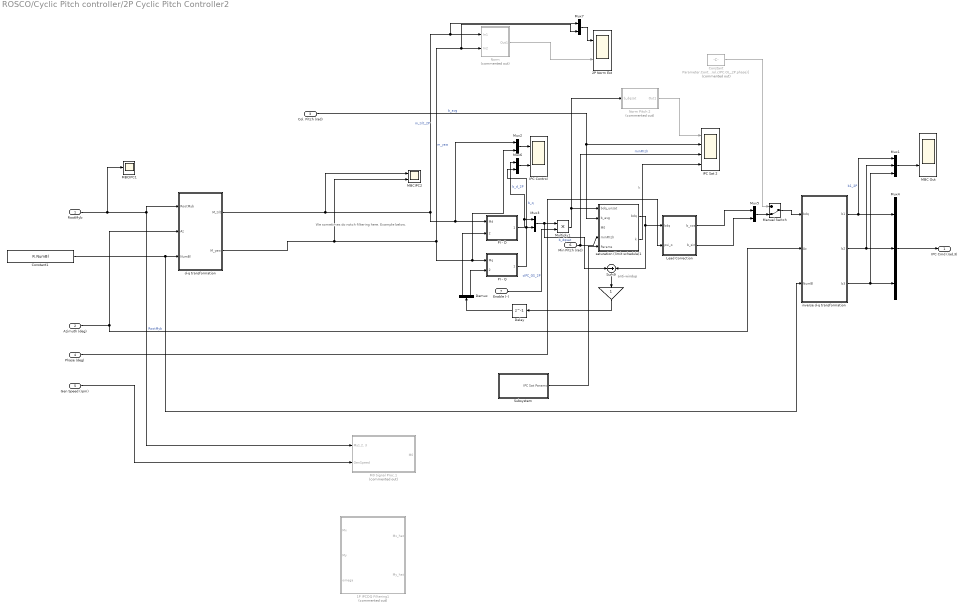
== system ROSCO/Cyclic Pitch controller/2P Cyclic Pitch Controller2 ==
  note: We sometimes do notch filtering here. Example below.
  note: anti-windup
  note: k
  RootMyb : Inport
  Azimuth (deg) : Inport  Port=2
  Col. Pitch (rad) : Inport  Port=3
  Phase (deg) : Inport  Port=4
  Gen Speed (rpm) : Inport  Port=5
  Min Pitch (rad) : Inport  Port=6
  Enable (-) : Inport  Port=7
  " " : Gain
  1P IPCDQ Filtering1 : Subsystem  Commented=on
  2P Norm Est : Scope  NumInputPorts=2
  Constant : Constant  Commented=on  Value=Parameter.Control.cIPC.OL_2P.amp * [cosd(Parameter.Control.cIPC.OL_2P.phase), sind(Parameter.Control.cIPC.OL_2P.phase)]
  Constant1 : Constant  Value=R.NumBl
  Delay : Delay  DelayLength=1
  Demux : Demux  Outputs=2
  IPC Control : Scope  NumInputPorts=2
  IPC Sat 2 : Scope  NumInputPorts=4
  Lead Correction : MATLAB Function  TreatAsAtomicUnit=on
  M0 Signal Proc.1 : Subsystem  Commented=on
  MBC Out : Scope  NumInputPorts=2
  MBCIPC1 : Scope
  MBCIPC2 : Scope  NumInputPorts=2
  Manual Switch : ManualSwitch  CurrentSetting=0
  Multiply1 : Product
  Mux1 : Mux  Inputs=3
  Mux{2..3,5..7} (5 alike) : Mux  Inputs=2
  Mux4 : Mux  Inputs=3
  Norm : Subsystem  Commented=on
  Norm Pitch 2 : Subsystem  Commented=on
  PI - D : Subsystem  TreatAsAtomicUnit=on  SystemSampleTime=simu.dt
      settings: MinAlgLoopOccurrences=on
  PI - Q : Subsystem  TreatAsAtomicUnit=on  SystemSampleTime=simu.dt
      settings: MinAlgLoopOccurrences=on
  Subsystem : Subsystem
  Sum9 : Sum  Inputs=-|+
  d-q transformation : MATLAB Function  TreatAsAtomicUnit=on
  inverse d-q transformation : MATLAB Function  TreatAsAtomicUnit=on
  saturation (limit schedule)1 : MATLAB Function  TreatAsAtomicUnit=on
  IPC Cmd (rad,3) : Outport  VectorParamsAs1DForOutWhenUnconnected=off
  wires:
  Enable (-)/1 -> Multiply1/2  "cIPC_GS_2P"
  Norm Pitch 2/1(Out1) -> IPC Sat 2/1
  Min Pitch (rad)/1 -> saturation (limit schedule)1/4(minPitch), IPC Sat 2/3  "minPitch"
  Norm/1(Out1) -> 2P Norm Est/2
  Mux7/1 -> 2P Norm Est/1
  Mux2/1 -> IPC Control/1
  Mux6/1 -> IPC Control/2
  Mux1/1 -> MBC Out/2
  d-q transformation/2(M_yaw) -> PI - Q/1(Mq), Mux2/2, Norm/2(In2), Mux7/2, MBCIPC2/2  "m_yaw"
  Constant1/1 -> inverse d-q transformation/3(NumBl), d-q transformation/3(NumBl)
  saturation (limit schedule)1/2(k) -> IPC Sat 2/4
  Lead Correction/2(b_sin) -> Mux5/2
  Lead Correction/1(b_cos) -> Mux5/1
  Azimuth (deg)/1 -> inverse d-q transformation/2(Az), d-q transformation/2(Az)
  Sum9/1 -> " "/1
  RootMyb/1 -> MBCIPC1/1, M0 Signal Proc.1/1("My1,2, 3"), d-q transformation/1(RootMyb)  "RootMyb"
  " "/1 -> Delay/1
  Delay/1 -> Demux/1
  Mux4/1 -> IPC Cmd (rad,3)/1
  inverse d-q transformation/2(b2) -> Mux4/2, Mux1/2
  Demux/2 -> PI - Q/2(Anti-windup)
  inverse d-q transformation/1(b1) -> Mux4/1, Mux1/1  "b1_2P"
  Demux/1 -> PI - D/2(Anti-windup)
  PI - D/1(Theta_tilt) -> Mux6/1, Mux3/1  "b_d_2P"
  PI - Q/1(Theta_yaw) -> Mux6/2, Mux3/2  "b_q"
  Phase (deg)/1 -> Lead Correction/2(psi_o)
  inverse d-q transformation/3(b3) -> Mux4/3, Mux1/3
  d-q transformation/1(M_tilt) -> PI - D/1(Md), Mux2/1, Norm/1(In1), Mux7/1, MBCIPC2/1  "m_tilt_2P"
  Gen Speed (rpm)/1 -> M0 Signal Proc.1/2(GenSpeed)
  saturation (limit schedule)1/1(bdq) -> Lead Correction/1(bdq), Sum9/2
  Col. Pitch (rad)/1 -> IPC Sat 2/2, saturation (limit schedule)1/2(b_avg)  "b_avg"
  Subsystem/1(IPC Sat Params) -> saturation (limit schedule)1/5(Params)
  Mux3/1 -> Sum9/1, Multiply1/1  "b_dqsat"
  Multiply1/1 -> Norm Pitch 2/1(b_dqsat), saturation (limit schedule)1/1(bdq_unsat)
  Mux5/1 -> Manual Switch/2
  Manual Switch/1 -> inverse d-q transformation/1(bdq)
  Constant/1 -> Manual Switch/1

== system ROSCO/Fl_PD/Integral ==
  x : Inport
  Gain : Inport  Port=2
  Gain1 : Gain  Gain=simu.dt
  Maximum Pitch : Constant  Value=100
  Minimum Pitch : Constant  Value=-100
  Multiply : Product
  Saturate Integral Term : simulink/Discontinuities/Saturation Dynamic  OutMin=[]  OutMax=[]  OutDataTypeStr=Inherit: Same as second input  OutDataType=fixdt(1, 16)  OutScaling=2^-10  RndMeth=Nearest  DoSatur=off
  Scope : Scope  NumInputPorts=2
  Sum : Sum  Inputs=|++
  Unit Delay : UnitDelay  SampleTime=-1  HasFrameUpgradeWarning=on
  Int x : Outport  VectorParamsAs1DForOutWhenUnconnected=off
  wires:
  Maximum Pitch/1 -> Saturate Integral Term/1
  Unit Delay/1 -> Sum/2
  Minimum Pitch/1 -> Saturate Integral Term/3
  Sum/1 -> Saturate Integral Term/2
  x/1 -> Scope/1, Gain1/1
  Gain/1 -> Multiply/2
  Saturate Integral Term/1 -> Scope/2, Int x/1, Unit Delay/1
  Gain1/1 -> Multiply/1
  Multiply/1 -> Sum/1

== system ROSCO/PitchSaturation/Integral ==
  x : Inport
  Gain : Inport  Port=2
  Gain1 : Gain  Gain=simu.dt
  Maximum Pitch : Constant  Value=100
  Minimum Pitch : Constant  Value=-100
  Multiply : Product
  Saturate Integral Term : simulink/Discontinuities/Saturation Dynamic  OutMin=[]  OutMax=[]  OutDataTypeStr=Inherit: Same as second input  OutDataType=fixdt(1, 16)  OutScaling=2^-10  RndMeth=Nearest  DoSatur=off
  Scope : Scope  NumInputPorts=2
  Sum : Sum  Inputs=|++
  Unit Delay : UnitDelay  SampleTime=-1  HasFrameUpgradeWarning=on
  Int x : Outport  VectorParamsAs1DForOutWhenUnconnected=off
  wires:
  Maximum Pitch/1 -> Saturate Integral Term/1
  Unit Delay/1 -> Sum/2
  Minimum Pitch/1 -> Saturate Integral Term/3
  Sum/1 -> Saturate Integral Term/2
  x/1 -> Scope/1, Gain1/1
  Gain/1 -> Multiply/2
  Saturate Integral Term/1 -> Scope/2, Int x/1, Unit Delay/1
  Gain1/1 -> Multiply/1
  Multiply/1 -> Sum/1

== system ROSCO/SetpointSmoother/Filter Delta_GenRef ==
  GainBias : Inport
  Discrete Filter : DiscreteFilter  Numerator=F.F_SS.b  Denominator=F.F_SS.a
  GainBiasF : Outport  VectorParamsAs1DForOutWhenUnconnected=off
  wires:
  Discrete Filter/1 -> GainBiasF/1
  GainBias/1 -> Discrete Filter/1

== system ROSCO/Torque Controller/Integral ==
  SpeedErr : Inport
  Gain : Inport  Port=2
  Gain1 : Gain  Gain=simu.dt
  Maximum Torque : Constant  Value=R.VS_RtTq
  Minimum Torque : Constant  Value=0
  Multiply : Product
  Saturate Integral Term : simulink/Discontinuities/Saturation Dynamic  OutMin=[]  OutMax=[]  OutDataTypeStr=Inherit: Same as second input  OutDataType=fixdt(1, 16)  OutScaling=2^-10  RndMeth=Nearest  DoSatur=off
  Sum : Sum  Inputs=|++
  Unit Delay : UnitDelay  InitialCondition=R.VS_RtTq  SampleTime=-1  HasFrameUpgradeWarning=on
  IntSpdErr : Outport  VectorParamsAs1DForOutWhenUnconnected=off
  wires:
  Maximum Torque/1 -> Saturate Integral Term/1
  Unit Delay/1 -> Sum/2
  Minimum Torque/1 -> Saturate Integral Term/3
  Sum/1 -> Saturate Integral Term/2
  SpeedErr/1 -> Gain1/1
  Gain/1 -> Multiply/2
  Saturate Integral Term/1 -> IntSpdErr/1, Unit Delay/1
  Gain1/1 -> Multiply/1
  Multiply/1 -> Sum/1

== system ROSCO/Torque Controller/VS_OmegaRef ==
  WindSpeedEst : Inport
  Omega_opt : Subsystem
  Reference TSR : Constant  Value=R.VS_TSRopt
  Saturation : Saturate  UpperLimit=R.PC_RefSpd  LowerLimit=R.VS_MinOMSpd
  To Workspace1 : ToWorkspace  VariableName=Om_opt  SaveFormat=Timeseries  SampleTime=-1
  VS_OmegaOpt : Outport  VectorParamsAs1DForOutWhenUnconnected=off
  wires:
  WindSpeedEst/1 -> Omega_opt/2(Wind Speed)
  Omega_opt/1(Omega_opt) -> Saturation/1
  Reference TSR/1 -> Omega_opt/1(TSR_opt)
  Saturation/1 -> VS_OmegaOpt/1, To Workspace1/1

== system ROSCO/Wind Speed Estimator/WE_Params ==
  Constant1 : Constant  Value=R.WE_Jtot
  Constant2 : Constant  Value=R.WE_RhoAir
  Constant3 : Constant  Value=R.WE_BladeRadius
  Constant4 : Constant  Value=R.WE_GearboxRatio
  Mux : Mux
  WE_Params : Outport
  wires:
  Constant2/1 -> Mux/2
  Mux/1 -> WE_Params/1
  Constant4/1 -> Mux/4
  Constant1/1 -> Mux/1
  Constant3/1 -> Mux/3

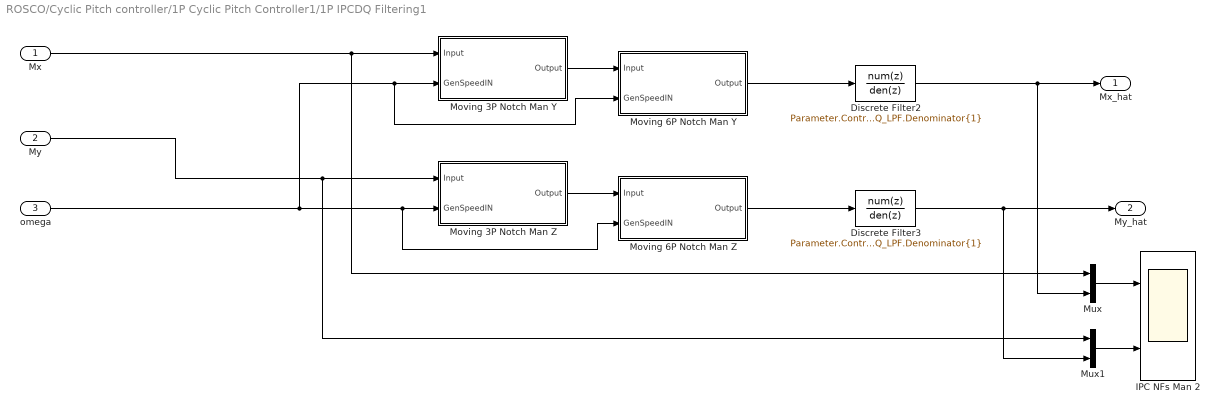
== system ROSCO/Cyclic Pitch controller/1P Cyclic Pitch Controller1/1P IPCDQ Filtering1 ==
  Mx : Inport
  My : Inport  Port=2
  omega : Inport  Port=3
  Discrete Filter2 : DiscreteFilter  Numerator=Parameter.Control.cIPC.IPCDQ_LPF.Numerator{1}  Denominator=Parameter.Control.cIPC.IPCDQ_LPF.Denominator{1}  SampleTime=Parameter.Control.DT
  Discrete Filter3 : DiscreteFilter  Numerator=Parameter.Control.cIPC.IPCDQ_LPF.Numerator{1}  Denominator=Parameter.Control.cIPC.IPCDQ_LPF.Denominator{1}  SampleTime=Parameter.Control.DT
  IPC NFs Man 2 : Scope  NumInputPorts=2
  Moving 3P Notch Man Y : Subsystem
  Moving 3P Notch Man Z : Subsystem
  Moving 6P Notch Man Y : Subsystem
  Moving 6P Notch Man Z : Subsystem
  Mux : Mux  Inputs=2
  Mux1 : Mux  Inputs=2
  Mx_hat : Outport  VectorParamsAs1DForOutWhenUnconnected=off
  My_hat : Outport  Port=2  VectorParamsAs1DForOutWhenUnconnected=off
  wires:
  omega/1 -> Moving 6P Notch Man Y/2(GenSpeedIN), Moving 3P Notch Man Y/2(GenSpeedIN), Moving 6P Notch Man Z/2(GenSpeedIN), Moving 3P Notch Man Z/2(GenSpeedIN)
  Mx/1 -> Mux/1, Moving 3P Notch Man Y/1(Input)
  My/1 -> Mux1/1, Moving 3P Notch Man Z/1(Input)
  Moving 6P Notch Man Z/1(Output) -> Discrete Filter3/1
  Moving 6P Notch Man Y/1(Output) -> Discrete Filter2/1
  Moving 3P Notch Man Y/1(Output) -> Moving 6P Notch Man Y/1(Input)
  Moving 3P Notch Man Z/1(Output) -> Moving 6P Notch Man Z/1(Input)
  Mux1/1 -> IPC NFs Man 2/2
  Mux/1 -> IPC NFs Man 2/1
  Discrete Filter3/1 -> Mux1/2, My_hat/1
  Discrete Filter2/1 -> Mux/2, Mx_hat/1

== system ROSCO/Cyclic Pitch controller/1P Cyclic Pitch Controller1/M0 Signal Proc.1 ==
  "My1,2, 3" : Inport
  GenSpeed : Inport  Port=2
  Add : Sum  Inputs=+++
  Demux1 : Demux  Outputs=3
  Discrete Filter : DiscreteFilter  Numerator=Parameter.Control.cIPC.PSM0_LPF.Numerator{1}  Denominator=Parameter.Control.cIPC.PSM0_LPF.Denominator{1}  a0EqualsOne=on
  Gain : Gain  Gain=1/3
  Moving 1P Notch Man : Subsystem
  Moving 3P Notch Man : Subsystem
  Mux : Mux  Inputs=2
  Scope : Scope  NumInputPorts=2
  M0 : Outport  VectorParamsAs1DForOutWhenUnconnected=off
  wires:
  Demux1/1 -> Add/1
  Demux1/2 -> Add/2
  Add/1 -> Gain/1
  "My1,2, 3"/1 -> Demux1/1
  GenSpeed/1 -> Moving 3P Notch Man/2(GenSpeedIN), Moving 1P Notch Man/2(GenSpeedIN)
  Demux1/3 -> Add/3
  Moving 1P Notch Man/1(Output) -> Moving 3P Notch Man/1(Input)
  Mux/1 -> Scope/2
  Gain/1 -> Scope/1, Moving 1P Notch Man/1(Input)
  Moving 3P Notch Man/1(Output) -> Discrete Filter/1
  Discrete Filter/1 -> Mux/1, M0/1

== system ROSCO/Cyclic Pitch controller/1P Cyclic Pitch Controller1/Norm ==
  In1 : Inport
  In2 : Inport  Port=2
  Add : Sum
  Discrete Filter1 : DiscreteFilter  Numerator=Parameter.Control.cIPC.IPCDQ_LPF.num{1}  Denominator=Parameter.Control.cIPC.IPCDQ_LPF.den{1}  SampleTime=Parameter.Control.DT
  Product : Product
  Product1 : Product
  Sqrt : Sqrt
  Out1 : Outport  VectorParamsAs1DForOutWhenUnconnected=off
  wires:
  Product/1 -> Add/1
  Product1/1 -> Add/2
  Sqrt/1 -> Discrete Filter1/1
  Add/1 -> Sqrt/1
  In2/1 -> Product1/1, Product1/2
  In1/1 -> Product/1, Product/2
  Discrete Filter1/1 -> Out1/1

== system ROSCO/Cyclic Pitch controller/1P Cyclic Pitch Controller1/Norm Pitch ==
  b_dqsat : Inport
  Demux1 : Demux  Outputs=2
  Sqrt : Sqrt
  Square : Math  Operator=square  SignedPower=on
  Square1 : Math  Operator=square  SignedPower=on
  Sum : Sum
  Out1 : Outport  VectorParamsAs1DForOutWhenUnconnected=off
  wires:
  Demux1/1 -> Square/1
  Square1/1 -> Sum/2
  b_dqsat/1 -> Demux1/1
  Sum/1 -> Sqrt/1
  Demux1/2 -> Square1/1
  Square/1 -> Sum/1
  Sqrt/1 -> Out1/1

== system ROSCO/Cyclic Pitch controller/1P Cyclic Pitch Controller1/PI - D ==
  Md : Inport
  Anti-windup : Inport  Port=2
  Discrete Derivative : simulink/Discrete/Discrete Derivative  gainval=1.0  ICPrevScaledInput=0.0  OutMin=[]  OutMax=[]  OutDataType=fixdt(1, 16)  OutScaling=2^-10  DoSatur=off
  Discrete Filter1 : DiscreteFilter  Commented=through  Numerator=Parameter.Control.cIPC.IPCDQ_LPF.num{1}  Denominator=Parameter.Control.cIPC.IPCDQ_LPF.den{1}  SampleTime=Parameter.Control.DT
  Integrator : DiscreteIntegrator  IntegratorMethod=Integration: Backward Euler  gainval=1  SampleTime=simu.dt  UpperSaturationLimit=1.570796/(.008068634/9.5492966)/(1./(1.+pi/2/.109997))  LowerSaturationLimit=0  ICPrevOutput=DiscIntNeverNeededParam  ICPrevScaledInput=DiscIntNeverNeededParam
  Kd : Gain  Gain=0
  Ki : Gain  Gain=R.IPC_KI_2P
  Kp : Gain  Gain=R.IPC_KP_1P
  Scope : Scope  NumInputPorts=2
  Sum3 : Sum  Inputs=+++
  Sum8 : Sum  Inputs=|++
  Theta_tilt : Outport  VectorParamsAs1DForOutWhenUnconnected=off
  wires:
  Ki/1 -> Sum8/1
  Sum3/1 -> Scope/1, Theta_tilt/1
  Md/1 -> Ki/1, Kp/1, Discrete Filter1/1
  Anti-windup/1 -> Scope/2, Sum8/2
  Sum8/1 -> Integrator/1
  Kd/1 -> Discrete Derivative/1
  Kp/1 -> Sum3/2
  Discrete Derivative/1 -> Sum3/1
  Integrator/1 -> Sum3/3
  Discrete Filter1/1 -> Kd/1

== system ROSCO/Cyclic Pitch controller/1P Cyclic Pitch Controller1/PI - Q ==
  Mq : Inport
  Anti-windup : Inport  Port=2
  Discrete Derivative : simulink/Discrete/Discrete Derivative  gainval=1.0  ICPrevScaledInput=0.0  OutMin=[]  OutMax=[]  OutDataType=fixdt(1, 16)  OutScaling=2^-10  DoSatur=off
  Discrete Filter1 : DiscreteFilter  Commented=through  Numerator=Parameter.Control.cIPC.IPCDQ_LPF.num{1}  Denominator=Parameter.Control.cIPC.IPCDQ_LPF.den{1}  SampleTime=Parameter.Control.DT
  Integrator1 : DiscreteIntegrator  IntegratorMethod=Integration: Backward Euler  gainval=1  SampleTime=simu.dt  UpperSaturationLimit=1.570796/(.008068634/9.5492966)/(1./(1.+pi/2/.109997))  LowerSaturationLimit=0  ICPrevOutput=DiscIntNeverNeededParam  ICPrevScaledInput=DiscIntNeverNeededParam
  Kd : Gain  Gain=0
  Ki : Gain  Gain=R.IPC_KI_1P
  Kp : Gain  Gain=R.IPC_KP_1P
  Sum10 : Sum  Inputs=|++
  Sum3 : Sum  Inputs=+++
  Theta_yaw : Outport  VectorParamsAs1DForOutWhenUnconnected=off
  wires:
  Sum3/1 -> Theta_yaw/1
  Sum10/1 -> Integrator1/1
  Anti-windup/1 -> Sum10/2
  Integrator1/1 -> Sum3/3
  Ki/1 -> Sum10/1
  Kp/1 -> Sum3/2
  Mq/1 -> Discrete Filter1/1, Kp/1, Ki/1
  Kd/1 -> Discrete Derivative/1
  Discrete Derivative/1 -> Sum3/1
  Discrete Filter1/1 -> Kd/1

== system ROSCO/Cyclic Pitch controller/1P Cyclic Pitch Controller1/Subsystem1 ==
  Constant3 : Constant  Value=2
  Constant4 : Constant  Value=0
  Constant5 : Constant  Value=0
  Mux : Mux  Inputs=3
  IPC Sat Params : Outport  VectorParamsAs1DForOutWhenUnconnected=off
  wires:
  Constant3/1 -> Mux/1
  Constant4/1 -> Mux/2
  Constant5/1 -> Mux/3
  Mux/1 -> IPC Sat Params/1

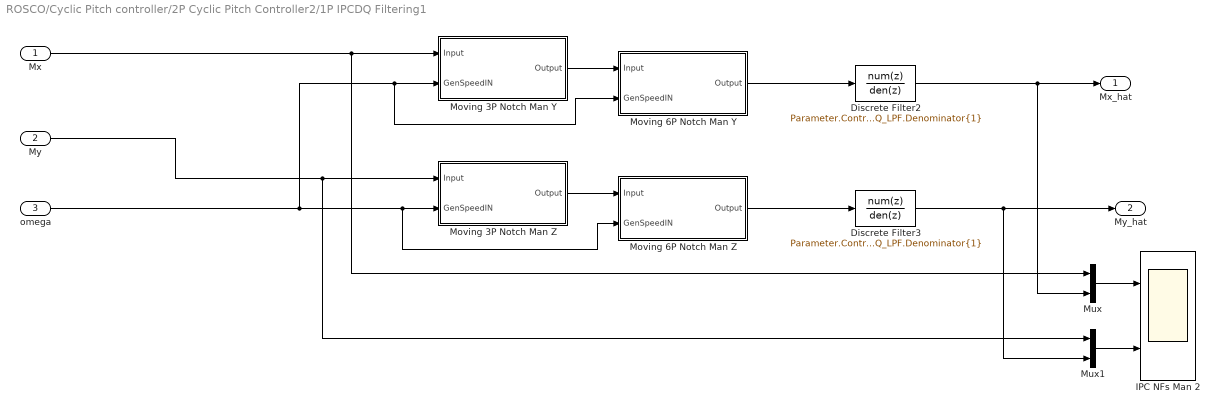
== system ROSCO/Cyclic Pitch controller/2P Cyclic Pitch Controller2/1P IPCDQ Filtering1 ==
  Mx : Inport
  My : Inport  Port=2
  omega : Inport  Port=3
  Discrete Filter2 : DiscreteFilter  Numerator=Parameter.Control.cIPC.IPCDQ_LPF.Numerator{1}  Denominator=Parameter.Control.cIPC.IPCDQ_LPF.Denominator{1}  SampleTime=Parameter.Control.DT
  Discrete Filter3 : DiscreteFilter  Numerator=Parameter.Control.cIPC.IPCDQ_LPF.Numerator{1}  Denominator=Parameter.Control.cIPC.IPCDQ_LPF.Denominator{1}  SampleTime=Parameter.Control.DT
  IPC NFs Man 2 : Scope  NumInputPorts=2
  Moving 3P Notch Man Y : Subsystem
  Moving 3P Notch Man Z : Subsystem
  Moving 6P Notch Man Y : Subsystem
  Moving 6P Notch Man Z : Subsystem
  Mux : Mux  Inputs=2
  Mux1 : Mux  Inputs=2
  Mx_hat : Outport  VectorParamsAs1DForOutWhenUnconnected=off
  My_hat : Outport  Port=2  VectorParamsAs1DForOutWhenUnconnected=off
  wires:
  omega/1 -> Moving 6P Notch Man Y/2(GenSpeedIN), Moving 3P Notch Man Y/2(GenSpeedIN), Moving 6P Notch Man Z/2(GenSpeedIN), Moving 3P Notch Man Z/2(GenSpeedIN)
  Mx/1 -> Mux/1, Moving 3P Notch Man Y/1(Input)
  My/1 -> Mux1/1, Moving 3P Notch Man Z/1(Input)
  Moving 6P Notch Man Z/1(Output) -> Discrete Filter3/1
  Moving 6P Notch Man Y/1(Output) -> Discrete Filter2/1
  Moving 3P Notch Man Y/1(Output) -> Moving 6P Notch Man Y/1(Input)
  Moving 3P Notch Man Z/1(Output) -> Moving 6P Notch Man Z/1(Input)
  Mux1/1 -> IPC NFs Man 2/2
  Mux/1 -> IPC NFs Man 2/1
  Discrete Filter3/1 -> Mux1/2, My_hat/1
  Discrete Filter2/1 -> Mux/2, Mx_hat/1

== system ROSCO/Cyclic Pitch controller/2P Cyclic Pitch Controller2/M0 Signal Proc.1 ==
  "My1,2, 3" : Inport
  GenSpeed : Inport  Port=2
  Add : Sum  Inputs=+++
  Demux1 : Demux  Outputs=3
  Discrete Filter : DiscreteFilter  Numerator=Parameter.Control.cIPC.PSM0_LPF.Numerator{1}  Denominator=Parameter.Control.cIPC.PSM0_LPF.Denominator{1}  a0EqualsOne=on
  Gain : Gain  Gain=1/3
  Moving 1P Notch Man : Subsystem
  Moving 3P Notch Man : Subsystem
  Mux : Mux  Inputs=2
  Scope : Scope  NumInputPorts=2
  M0 : Outport  VectorParamsAs1DForOutWhenUnconnected=off
  wires:
  Demux1/1 -> Add/1
  Demux1/2 -> Add/2
  Add/1 -> Gain/1
  "My1,2, 3"/1 -> Demux1/1
  GenSpeed/1 -> Moving 3P Notch Man/2(GenSpeedIN), Moving 1P Notch Man/2(GenSpeedIN)
  Demux1/3 -> Add/3
  Moving 1P Notch Man/1(Output) -> Moving 3P Notch Man/1(Input)
  Mux/1 -> Scope/2
  Gain/1 -> Scope/1, Moving 1P Notch Man/1(Input)
  Moving 3P Notch Man/1(Output) -> Discrete Filter/1
  Discrete Filter/1 -> Mux/1, M0/1

== system ROSCO/Cyclic Pitch controller/2P Cyclic Pitch Controller2/Norm ==
  In1 : Inport
  In2 : Inport  Port=2
  Add : Sum
  Discrete Filter1 : DiscreteFilter  Numerator=Parameter.Control.cIPC.IPCDQ_LPF.num{1}  Denominator=Parameter.Control.cIPC.IPCDQ_LPF.den{1}  SampleTime=Parameter.Control.DT
  Product : Product
  Product1 : Product
  Sqrt : Sqrt
  Out1 : Outport  VectorParamsAs1DForOutWhenUnconnected=off
  wires:
  Discrete Filter1/1 -> Out1/1
  In1/1 -> Product/2, Product/1
  In2/1 -> Product1/2, Product1/1
  Add/1 -> Sqrt/1
  Sqrt/1 -> Discrete Filter1/1
  Product1/1 -> Add/2
  Product/1 -> Add/1

== system ROSCO/Cyclic Pitch controller/2P Cyclic Pitch Controller2/Norm Pitch 2 ==
  b_dqsat : Inport
  Demux1 : Demux  Outputs=2
  Sqrt : Sqrt
  Square : Math  Operator=square  SignedPower=on
  Square1 : Math  Operator=square  SignedPower=on
  Sum : Sum
  Out1 : Outport  VectorParamsAs1DForOutWhenUnconnected=off
  wires:
  Sqrt/1 -> Out1/1
  Square/1 -> Sum/1
  Demux1/2 -> Square1/1
  Sum/1 -> Sqrt/1
  b_dqsat/1 -> Demux1/1
  Square1/1 -> Sum/2
  Demux1/1 -> Square/1

== system ROSCO/Cyclic Pitch controller/2P Cyclic Pitch Controller2/PI - D ==
  Md : Inport
  Anti-windup : Inport  Port=2
  Discrete Derivative : simulink/Discrete/Discrete Derivative  gainval=1.0  ICPrevScaledInput=0.0  OutMin=[]  OutMax=[]  OutDataType=fixdt(1, 16)  OutScaling=2^-10  DoSatur=off
  Discrete Filter1 : DiscreteFilter  Commented=through  Numerator=Parameter.Control.cIPC.IPCDQ_LPF.num{1}  Denominator=Parameter.Control.cIPC.IPCDQ_LPF.den{1}  SampleTime=Parameter.Control.DT
  Integrator : DiscreteIntegrator  IntegratorMethod=Integration: Backward Euler  gainval=1  SampleTime=simu.dt  UpperSaturationLimit=1.570796/(.008068634/9.5492966)/(1./(1.+pi/2/.109997))  LowerSaturationLimit=0  ICPrevOutput=DiscIntNeverNeededParam  ICPrevScaledInput=DiscIntNeverNeededParam
  Kd : Gain  Gain=0
  Ki : Gain  Gain=R.IPC_KI_2P
  Kp : Gain  Gain=R.IPC_KP_2P
  Sum3 : Sum  Inputs=+++
  Sum8 : Sum  Inputs=|++
  Theta_tilt : Outport  VectorParamsAs1DForOutWhenUnconnected=off
  wires:
  Discrete Filter1/1 -> Kd/1
  Integrator/1 -> Sum3/3
  Discrete Derivative/1 -> Sum3/1
  Kp/1 -> Sum3/2
  Kd/1 -> Discrete Derivative/1
  Sum8/1 -> Integrator/1
  Anti-windup/1 -> Sum8/2
  Md/1 -> Discrete Filter1/1, Kp/1, Ki/1
  Sum3/1 -> Theta_tilt/1
  Ki/1 -> Sum8/1

== system ROSCO/Cyclic Pitch controller/2P Cyclic Pitch Controller2/PI - Q ==
  Mq : Inport
  Anti-windup : Inport  Port=2
  Discrete Derivative : simulink/Discrete/Discrete Derivative  gainval=1.0  ICPrevScaledInput=0.0  OutMin=[]  OutMax=[]  OutDataType=fixdt(1, 16)  OutScaling=2^-10  DoSatur=off
  Discrete Filter1 : DiscreteFilter  Commented=through  Numerator=Parameter.Control.cIPC.IPCDQ_LPF.num{1}  Denominator=Parameter.Control.cIPC.IPCDQ_LPF.den{1}  SampleTime=Parameter.Control.DT
  Integrator1 : DiscreteIntegrator  IntegratorMethod=Integration: Backward Euler  gainval=1  SampleTime=simu.dt  UpperSaturationLimit=1.570796/(.008068634/9.5492966)/(1./(1.+pi/2/.109997))  LowerSaturationLimit=0  ICPrevOutput=DiscIntNeverNeededParam  ICPrevScaledInput=DiscIntNeverNeededParam
  Kd : Gain  Gain=0
  Ki : Gain  Gain=R.IPC_KI_2P
  Kp : Gain  Gain=R.IPC_KP_2P
  Sum10 : Sum  Inputs=|++
  Sum3 : Sum  Inputs=+++
  Theta_yaw : Outport  VectorParamsAs1DForOutWhenUnconnected=off
  wires:
  Discrete Filter1/1 -> Kd/1
  Discrete Derivative/1 -> Sum3/1
  Kd/1 -> Discrete Derivative/1
  Mq/1 -> Ki/1, Kp/1, Discrete Filter1/1
  Kp/1 -> Sum3/2
  Ki/1 -> Sum10/1
  Integrator1/1 -> Sum3/3
  Anti-windup/1 -> Sum10/2
  Sum10/1 -> Integrator1/1
  Sum3/1 -> Theta_yaw/1

== system ROSCO/Cyclic Pitch controller/2P Cyclic Pitch Controller2/Subsystem ==
  Constant3 : Constant  Value=2
  Constant4 : Constant  Value=0
  Constant5 : Constant  Value=0
  Mux : Mux  Inputs=3
  IPC Sat Params : Outport  VectorParamsAs1DForOutWhenUnconnected=off
  wires:
  Constant3/1 -> Mux/1
  Constant4/1 -> Mux/2
  Constant5/1 -> Mux/3
  Mux/1 -> IPC Sat Params/1

== system ROSCO/Torque Controller/VS_OmegaRef/Omega_opt ==
  note: % Assuming known wind speed, initially, and not using GenSpeed
  TSR_opt : Inport
  Wind Speed : Inport  Port=2
  Divide : Product  Inputs=*/
  Multiply : Product
  "Rot -> GenSpeed" : Gain  Gain=R.GBRatio
  Rotor Radius : Constant  Value=R.RotorRad
  Omega_opt : Outport  VectorParamsAs1DForOutWhenUnconnected=off
  wires:
  TSR_opt/1 -> Multiply/1
  Wind Speed/1 -> Multiply/2
  Multiply/1 -> Divide/1
  Rotor Radius/1 -> Divide/2
  Divide/1 -> "Rot -> GenSpeed"/1
  "Rot -> GenSpeed"/1 -> Omega_opt/1
